simulink model "quadrotor_2021b_06112024_Spring"  (R2023a)
settings: Solver=VariableStepAuto  StartTime=0.0  StopTime=40  RelTol=1e-3
InitFcn:
  | % quadrotor parameters
  | m = 1;
  | C = 1;
  | J_phi = 1;
  | l = 1;
  | J_theta = 1;
  | J_psi = 1;
  | M = blkdiag(1/m,C/J_phi,l/J_theta,l/J_psi);
  | g = 9.81;
  | 
  | % controller parameters
  | kappa = 200;
  | a_1 = 5;
  | a_2 = 10;
  | a_3 = 10;
  | a_4 = 5;
  | a_5 = 1;
  | 
  | ww=1;
  | gamma_1 = ww^4;
  | gamma_2 = 3*ww^3;
  | gamma_3 = 5*ww^2;
  | gamma_4 = 3*ww;
  | L = 5;
  | 
  | ell = 0.9;
settings Model: Creator=olegborisov  LastModifiedBy=Dell
settings SolverCC: ZeroCrossAlgorithm=Adaptive
settings DebuggingCC: IgnoredZcDiagnostic=none

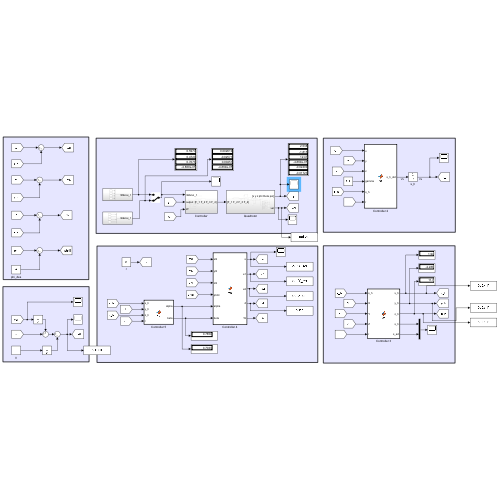
[thumbnail: Simulink's stored preview of the top-level diagram]
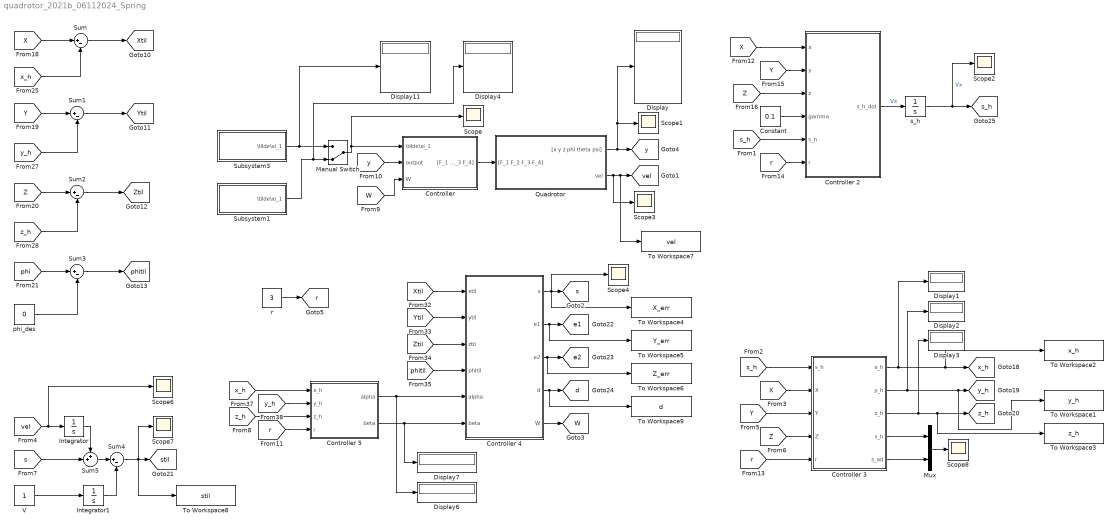
== system quadrotor_2021b_06112024_Spring ==
  Constant : Constant  Value=0.1
  Controller : Subsystem
  Controller 2 : MATLAB Function  TreatAsAtomicUnit=on
  Controller 3 : MATLAB Function  TreatAsAtomicUnit=on
  Controller 4 : MATLAB Function  TreatAsAtomicUnit=on
  Controller 5 : MATLAB Function  TreatAsAtomicUnit=on
  Display{,1..4,6..7,11} (8 alike) : Display
  Integrator : Integrator
  Integrator1 : Integrator
  Manual Switch : ManualSwitch  CurrentSetting=0
  Mux : Mux  Inputs=2
  Quadrotor : Subsystem
  Scope{,1..4,6..8} (8 alike) : Scope
  Subsystem1 : Subsystem
  Subsystem3 : Subsystem
  Sum{,1..4} (5 alike) : Sum  Inputs=|+-
  Sum5 : Sum  Inputs=++|
  To Workspace1 : ToWorkspace  VariableName=y_h  SaveFormat=Timeseries  SampleTime=-1
  To Workspace2 : ToWorkspace  VariableName=x_h  SaveFormat=Timeseries  SampleTime=-1
  To Workspace3 : ToWorkspace  VariableName=z_h  SaveFormat=Timeseries  SampleTime=-1
  To Workspace4 : ToWorkspace  VariableName=X_err  SaveFormat=Timeseries  SampleTime=-1
  To Workspace5 : ToWorkspace  VariableName=Y_err  SaveFormat=Timeseries  SampleTime=-1
  To Workspace6 : ToWorkspace  VariableName=Z_err  SaveFormat=Timeseries  SampleTime=-1
  To Workspace7 : ToWorkspace  VariableName=vel  SaveFormat=Timeseries  SampleTime=-1
  To Workspace8 : ToWorkspace  VariableName=stil  SaveFormat=Timeseries  SampleTime=-1
  To Workspace9 : ToWorkspace  VariableName=d  SaveFormat=Timeseries  SampleTime=-1
  V : Constant
  phi_des : Constant  Value=0
  r : Constant  Value=3
  s_h : Integrator
  tag scope: W=global, Xtil=global, Ytil=global, Ztil=global, d=global, e1=global, e2=global, phitil=global, r=global, s=global, s_h=global, stil=global, vel=global, x_h=global, y=global, y_h=global, z_h=global
  wires:
  Quadrotor/1("[x y z phi theta psi]") -> Display/1, Scope1/1, [y]
  Manual Switch/1 -> Scope/1, Controller/1(\tilde\xi_1)
  [Z] -> Controller 2/3(z)
  [Y] -> Controller 2/2(y)
  Constant/1 -> Controller 2/4(gamma)
  [X] -> Controller 2/1(x)
  Controller 4/2(e1) -> To Workspace5/1, [e1]
  Controller 5/2(beta) -> Controller 4/6(beta), Display7/1
  [Xtil] -> Controller 4/1(xtil)
  Controller 5/1(alpha) -> Display6/1, Controller 4/5(alpha)
  [y_h] -> Controller 5/2(y_h)
  [phitil] -> Controller 4/4(phitil)
  Controller 4/3(e2) -> To Workspace6/1, [e2]
  [x_h] -> Controller 5/1(x_h)
  Controller 4/4(d) -> To Workspace9/1, [d]
  [Ztil] -> Controller 4/3(ztil)
  [Ytil] -> Controller 4/2(ytil)
  [y_h] -> Sum1/2
  Sum1/1 -> [Ytil]
  Sum3/1 -> [phitil]
  [x_h] -> Sum/2
  phi_des/1 -> Sum3/2
  [z_h] -> Sum2/2
  [phi] -> Sum3/1
  [Y] -> Sum1/1
  Sum/1 -> [Xtil]
  Sum2/1 -> [Ztil]
  [Z] -> Sum2/1
  [X] -> Sum/1
  Controller/1("[F_1 F_2 F_3 F_4]") -> Quadrotor/1("[F_1 F_2 F_3 F_4]")
  Quadrotor/2(vel) -> To Workspace7/1, [vel], Scope3/1
  Sum4/1 -> To Workspace8/1, Scope7/1, [stil]
  Subsystem3/1(\tilde\xi_1) -> Manual Switch/1, Display11/1
  Controller 2/1(s_h_dot) -> s_h/1  "Vx"
  Controller 4/1(s) -> Scope4/1, To Workspace4/1, [s]
  s_h/1 -> Scope2/1, [s_h]  "Vx"
  [vel] -> Scope6/1, Integrator/1
  Integrator1/1 -> Sum4/2
  Subsystem1/1(\tilde\xi_1) -> Display4/1, Manual Switch/2
  [s_h] -> Controller 2/5(s_h)
  [z_h] -> Controller 5/3(z_h)
  Integrator/1 -> Sum5/1
  Sum5/1 -> Sum4/1
  [s] -> Sum5/2
  Controller 4/5(W) -> [W]
  [W] -> Controller/3(W)
  [X] -> Controller 3/2(X)
  [Y] -> Controller 3/3(Y)
  Controller 3/3(z_h) -> To Workspace3/1, [z_h], Display3/1
  Controller 3/1(x_h) -> Display1/1, To Workspace2/1, [x_h]
  [s_h] -> Controller 3/1("s_h ")
  [Z] -> Controller 3/4(Z)
  Mux/1 -> Scope8/1
  Controller 3/5(s_ad) -> Mux/2
  Controller 3/4(s_h) -> Mux/1
  Controller 3/2(y_h) -> Display2/1, To Workspace1/1, [y_h]
  V/1 -> Integrator1/1
  [y] -> Controller/2(output)
  [r] -> Controller 5/4(r)
  [r] -> Controller 3/5(r)
  [r] -> Controller 2/6(r)
  r/1 -> [r]

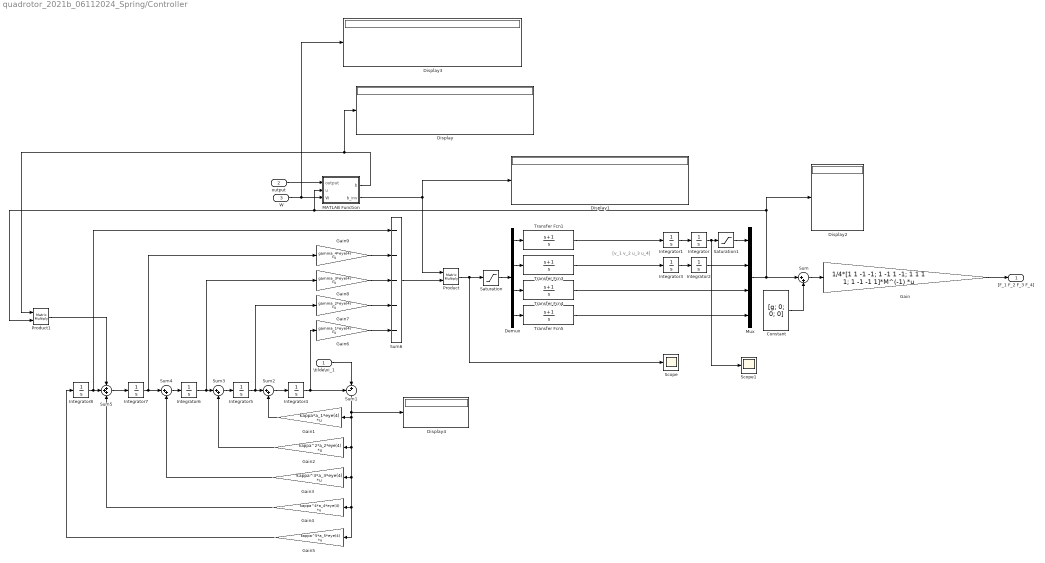
== system quadrotor_2021b_06112024_Spring/Controller ==
  note: [v_1 v_2 u_3 u_4]
  \tilde\xi_1 : Inport
  output : Inport  Port=2
  W : Inport  Port=3
  Constant : Constant  Value=[g; 0; 0; 0]  VectorParams1D=off
  Demux : Demux
  Display{,1..4} (5 alike) : Display
  Gain : Gain  Gain=1/4*[1 1 -1 -1; 1 -1 1 -1; 1 1 1 1; 1 -1 -1 1]*M^(-1)  Multiplication=Matrix(K*u) (u vector)
  Gain1 : Gain  Gain=kappa*a_1*eye(4)  Multiplication=Matrix(K*u) (u vector)
  Gain2 : Gain  Gain=kappa^2*a_2*eye(4)  Multiplication=Matrix(K*u) (u vector)
  Gain3 : Gain  Gain=kappa^3*a_3*eye(4)  Multiplication=Matrix(K*u) (u vector)
  Gain4 : Gain  Gain=kappa^4*a_4*eye(4)  Multiplication=Matrix(K*u) (u vector)
  Gain5 : Gain  Gain=kappa^5*a_5*eye(4)  Multiplication=Matrix(K*u) (u vector)
  Gain6 : Gain  Gain=gamma_1*eye(4)  Multiplication=Matrix(K*u) (u vector)
  Gain7 : Gain  Gain=gamma_2*eye(4)  Multiplication=Matrix(K*u) (u vector)
  Gain8 : Gain  Gain=gamma_3*eye(4)  Multiplication=Matrix(K*u) (u vector)
  Gain9 : Gain  Gain=gamma_4*eye(4)  Multiplication=Matrix(K*u) (u vector)
  Integrator{,1..8} (9 alike) : Integrator
  MATLAB Function : MATLAB Function  TreatAsAtomicUnit=on
  Mux : Mux
  Product : Product  Multiplication=Matrix(*)
  Product1 : Product  Multiplication=Matrix(*)
  Saturation : Saturate  UpperLimit=L  LowerLimit=-L
  Saturation1 : Saturate  UpperLimit=ell*g  LowerLimit=-ell*g
  Scope : Scope
  Scope1 : Scope
  Sum{,2..4} (4 alike) : Sum  Inputs=|++
  Sum1 : Sum  Inputs=-+|
  Sum5 : Sum  Inputs=+++
  Sum6 : Sum  Inputs=-----
  Transfer Fcn{1,3..5} (4 alike) : TransferFcn  Numerator=[1 1]  Denominator=[1 0]
  "[F_1 F_2 F_3 F_4]" : Outport
  wires:
  Gain/1 -> "[F_1 F_2 F_3 F_4]"/1
  Sum/1 -> Gain/1
  Constant/1 -> Sum/2
  Integrator1/1 -> Integrator/1
  Integrator3/1 -> Integrator2/1
  Integrator/1 -> Scope1/1, Saturation1/1
  Integrator2/1 -> Mux/2
  Mux/1 -> Display2/1, Product1/2, MATLAB Function/2(u), Sum/1
  Integrator4/1 -> Sum1/1, Gain6/1
  \tilde\xi_1/1 -> Sum1/2
  Sum1/1 -> Gain5/1, Gain4/1, Gain3/1, Gain2/1, Gain1/1, Display4/1
  Gain1/1 -> Sum2/2
  Sum2/1 -> Integrator4/1
  Sum3/1 -> Integrator5/1
  Gain2/1 -> Sum3/2
  Integrator6/1 -> Gain8/1, Sum3/1
  Sum4/1 -> Integrator6/1
  Gain3/1 -> Sum4/2
  Integrator7/1 -> Gain9/1, Sum4/1
  Sum5/1 -> Integrator7/1
  Gain4/1 -> Sum5/3
  Integrator8/1 -> Sum6/1, Sum5/2
  Gain5/1 -> Integrator8/1
  Gain6/1 -> Sum6/5
  Gain7/1 -> Sum6/4
  Gain8/1 -> Sum6/3
  Gain9/1 -> Sum6/2
  Sum6/1 -> Product/2
  Product/1 -> Scope/1, Saturation/1
  Product1/1 -> Sum5/1
  MATLAB Function/2(b_inv) -> Display1/1, Product/1
  MATLAB Function/1(b) -> Product1/1, Display/1
  output/1 -> MATLAB Function/1(output)
  Saturation1/1 -> Mux/1
  W/1 -> Display3/1, MATLAB Function/3(W)
  Saturation/1 -> Demux/1
  Demux/1 -> Transfer Fcn1/1
  Demux/2 -> Transfer Fcn3/1
  Demux/3 -> Transfer Fcn4/1
  Transfer Fcn4/1 -> Mux/3
  Demux/4 -> Transfer Fcn5/1
  Integrator5/1 -> Gain7/1, Sum2/1
  Transfer Fcn1/1 -> Integrator1/1
  Transfer Fcn3/1 -> Integrator3/1
  Transfer Fcn5/1 -> Mux/4

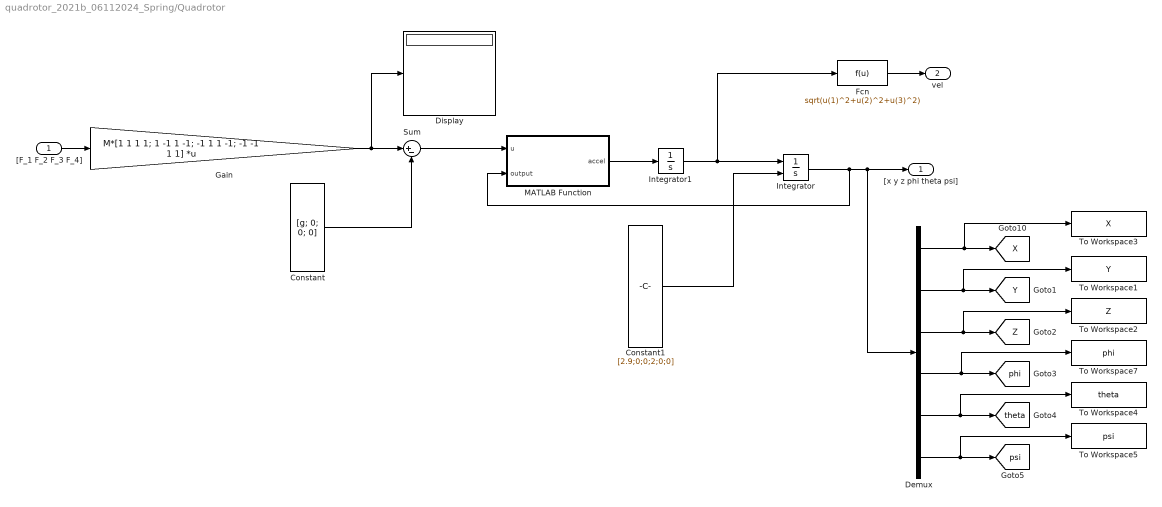
== system quadrotor_2021b_06112024_Spring/Quadrotor ==
  "[F_1 F_2 F_3 F_4]" : Inport
  Constant : Constant  Value=[g; 0; 0; 0]  VectorParams1D=off
  Constant1 : Constant  Value=[2.9;0;0;2;0;0]  VectorParams1D=off
  Demux : Demux  Outputs=6
  Display : Display
  Fcn : Fcn  Expr=sqrt(u(1)^2+u(2)^2+u(3)^2)
  Gain : Gain  Gain="M*[1 1 1 1; 1 -1 1 -1; -1 1 1 -1;  -1 -1 1 1]"  Multiplication=Matrix(K*u) (u vector)
  Integrator : Integrator  InitialConditionSource=external  InitialCondition=[0;1;1;1;0;0]
  Integrator1 : Integrator
  MATLAB Function : MATLAB Function  TreatAsAtomicUnit=on
  Sum : Sum  Inputs=|+-
  To Workspace1 : ToWorkspace  VariableName=Y  SaveFormat=Timeseries  SampleTime=-1
  To Workspace2 : ToWorkspace  VariableName=Z  SaveFormat=Timeseries  SampleTime=-1
  To Workspace3 : ToWorkspace  VariableName=X  SaveFormat=Timeseries  SampleTime=-1
  To Workspace4 : ToWorkspace  VariableName=theta  SaveFormat=Timeseries  SampleTime=-1
  To Workspace5 : ToWorkspace  VariableName=psi  SaveFormat=Timeseries  SampleTime=-1
  To Workspace7 : ToWorkspace  VariableName=phi  SaveFormat=Timeseries  SampleTime=-1
  "[x y z phi theta psi]" : Outport
  vel : Outport  Port=2
  tag scope: X=global, Y=global, Z=global, phi=global, psi=global, theta=global
  wires:
  Integrator1/1 -> Fcn/1, Integrator/1
  Integrator/1 -> Demux/1, "[x y z phi theta psi]"/1, MATLAB Function/2(output)
  MATLAB Function/1(accel) -> Integrator1/1
  "[F_1 F_2 F_3 F_4]"/1 -> Gain/1
  Gain/1 -> Display/1, Sum/1
  Constant/1 -> Sum/2
  Sum/1 -> MATLAB Function/1(u)
  Constant1/1 -> Integrator/2
  Demux/1 -> To Workspace3/1, [X]
  Demux/2 -> To Workspace1/1, [Y]
  Demux/3 -> To Workspace2/1, [Z]
  Demux/4 -> To Workspace7/1, [phi]
  Demux/5 -> To Workspace4/1, [theta]
  Demux/6 -> To Workspace5/1, [psi]
  Fcn/1 -> vel/1

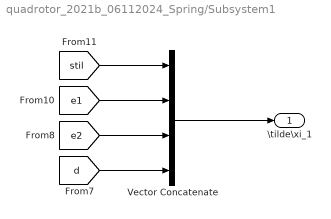
== system quadrotor_2021b_06112024_Spring/Subsystem1 ==
  Vector Concatenate : Concatenate  NumInputs=4
  \tilde\xi_1 : Outport
  wires:
  [e1] -> Vector Concatenate/2
  [stil] -> Vector Concatenate/1
  [e2] -> Vector Concatenate/3
  Vector Concatenate/1 -> \tilde\xi_1/1
  [d] -> Vector Concatenate/4

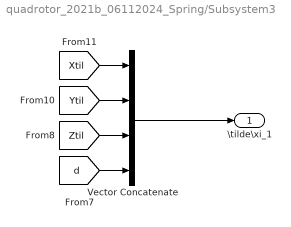
== system quadrotor_2021b_06112024_Spring/Subsystem3 ==
  Vector Concatenate : Concatenate  NumInputs=4
  \tilde\xi_1 : Outport
  wires:
  Vector Concatenate/1 -> \tilde\xi_1/1
  [Ztil] -> Vector Concatenate/3
  [d] -> Vector Concatenate/4
  [Ytil] -> Vector Concatenate/2
  [Xtil] -> Vector Concatenate/1

== matlab function quadrotor_2021b_06112024_Spring/Controller/MATLAB Function ==
  data: output input; u input; b output; b_inv output; W input
function [b,b_inv] = fcn(output,u,W)

no = 0;
simple = 1;
full = 2;

flag = full;

phi = output(4);

theta = output(5);

psi = output(6);

ct = cos(theta);
st = sin(theta);

cp = cos(psi);
sp = sin(psi);

g = 9.81;
dd = u(1)+g;

%W=W^(-1);

b = W*[cos(phi) -sin(phi) 0 0; 
     sin(phi) cos(phi) 0 0; 
     0 0 1 0; 
     0 0 0 1]*...
    [st*cp 0 ct*cp*dd -st*sp*dd; 
     -sp 0 0 -cp*dd;
     ct*cp 0 -st*cp*dd -ct*sp*dd;
     0 1 0 0];
b_inv  = inv(b);

== matlab function quadrotor_2021b_06112024_Spring/Quadrotor/MATLAB Function ==
  data: u input; accel output; output input
function accel = fcn(u, output)

g = 9.81;
phi = output(4);
theta = output(5);
psi = output(6);

accel_lin = [cos(phi)*sin(theta)*cos(psi)+sin(phi)*sin(psi);...
    sin(phi)*sin(theta)*cos(psi)-cos(phi)*sin(psi);...
    cos(theta)*cos(psi)]*(u(1)+g)-[0; 0; g];

accel_ang = [u(2); u(3); u(4)];

accel = [accel_lin; accel_ang];

== matlab function quadrotor_2021b_06112024_Spring/Controller 2 ==
  data: x input; y input; z input; gamma input; s_h_dot output; s_h input; r input
function s_h_dot   = fcn(x,y,z,gamma,s_h,r)


% Прямые x+y = 0 и x+z = 0
%H = 3*s_h - x - y - z;

% Спираль


rho = sign(1 + r*cos(s_h)*x + r*sin(s_h)*y);

H = r*sin(s_h)*x - r*cos(s_h)*y - z + s_h;

s_h_dot = -gamma*rho*H;

== matlab function quadrotor_2021b_06112024_Spring/Controller 3 ==
  data: s_h input; x_h output; y_h output; z_h output; s_h output; X input; Y input; Z input; s_ad output; r input
function [x_h,y_h,z_h,s_h,s_ad]   = fcn(s_h, X,Y,Z,r)

s_ad = s_h;

% если кривая, то можно использовать исходный s_h


% если прямая, то можно раскомментировать следующую строку
s_h = 1/3*(X+Y+Z);



% если прямая точно известная, то использовать эти 4 формулы, если кривая,
% то надо закомментировать и использовать блок ниже


% x_h = s_h;
% 
% y_h = s_h;
% 
% z_h = s_h;


% если кривая (гнапример спираль), то раскомментировать этот блок


x_h = r * cos(s_ad);

y_h = r* sin(s_ad);

z_h = s_ad;

== matlab function quadrotor_2021b_06112024_Spring/Controller 4 ==
  data: s output; xtil input; ytil input; ztil input; phitil input; alpha input; beta input; e1 output; e2 output; d output; W output
function [s, e1,e2,d, W]   = fcn(xtil,ytil,ztil,phitil,alpha,beta)

xyzphitil = [xtil;ytil;ztil;phitil];


W=  [cos(beta) 0 sin(beta) 0; 0 1 0 0; -sin(beta) 0 cos(beta) 0; 0 0 0 1]*...
    [cos(alpha) sin(alpha) 0 0; -sin(alpha) cos(alpha) 0 0;  0 0 1 0; 0 0 0 1];


P = W*xyzphitil;

s = P(1);

e1 = P(2);

e2 = P(3);

d = P(4);

zeta =[s;e1;e2;d];

== matlab function quadrotor_2021b_06112024_Spring/Controller 5 ==
  data: x_h input; y_h input; alpha output; beta output; z_h input; r input
function [alpha,beta]   = fcn(x_h,y_h,z_h,r)


% atna2(sin *, cos *)

% cos alpha = d varphi_xy / dy;  
% sin alpha = -d varphi_xy / dx;

% cos beta = d varphi_xz / dz;  
% sin beta = -d varphi_xz / dx;


% Прямые x+y = 0 и x+z = 0

alpha = atan2(-(-1), 1);

beta = atan2(-(-1), 1);


% Спираль


alpha = atan2(x_h, -y_h);

beta = atan2(1, 1);
